simulink model "MPC_mobile_base_KIN_IPOPT_fast_ROS"  (R2018b)
settings: Solver=ode4  StartTime=0.0  StopTime=inf  FixedStep=Tsample  RelTol=1e-3
values from neighbouring files (symbols this model uses):
  initialize_starting_point = 1    [init_prova_vera1.mat]    (also in init_prova_vera3.mat; prova_vera1.mat = 0; prova_vera2.mat = 0)
  N = length(q)    [FK.m]    (also in FK_generation.m = size(DHTABLE,1); init_prova_vera1.mat = 10; init_prova_vera3.mat = 10; jacobian_MM.m)
  Np = 18    [init_prova_vera1.mat]    (also in init_prova_vera3.mat; initialization.m = Lf*2 + Lp*6; prova_vera1.mat; prova_vera2.mat)
  T = cell(N+1,1)    [FK.m]    (also in init_prova_vera1.mat = 0.5; init_prova_vera3.mat = 0.5; jacobian_MM.m; matlabultimo.mat = 0.5)
  Tsample = 0.01    [init_prova_vera1.mat]    (also in init_prova_vera3.mat; matlabultimo.mat; prova_vera1.mat; prova_vera2.mat)
  xd = [0 0 0 0 0 0 0 0 0 0.0238792670666 0.415141969475 1.22261425872 ... (1458 elements, 18x81)]    [init_prova_vera1.mat]    (also in init_prova_vera3.mat; liveplot.m = evalin('base','xd'); matlabultimo.mat = [0 0 0 0 0 0 0 0 0 -0.528285242967 -0.106449885857 1.3372295; prova_vera1.mat)
undefined symbols (not defined in the file or in its folder): Angular, Linear
libraries: robotlib x6, simulink x6, dspstat3 x3, peGeneralControl x1, sharedtransform x1
settings Model: EnablePacing=on  Creator=francesco  LastModifiedBy=francesco
settings ModelReferenceCC: PropagateVarSize=Only when enabling

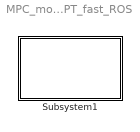
== system MPC_mobile_base_KIN_IPOPT_fast_ROS ==
  Subsystem1 : Subsystem  InitFcn=initialization

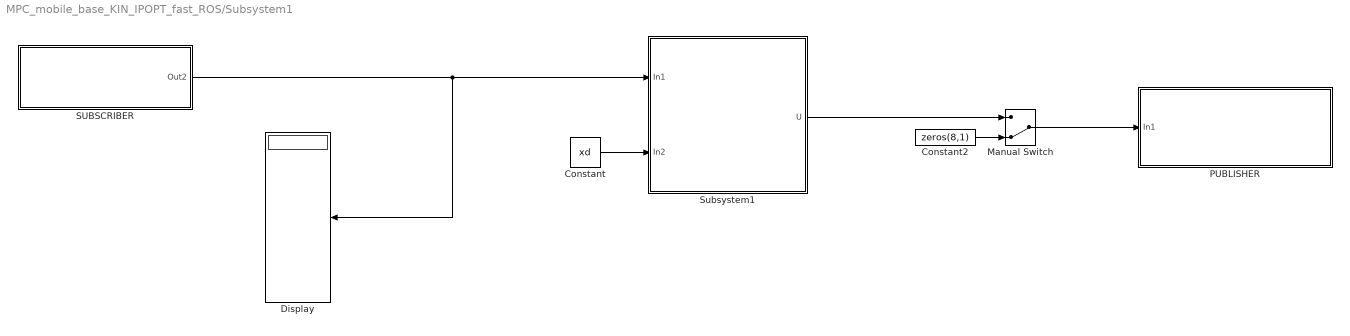
== system MPC_mobile_base_KIN_IPOPT_fast_ROS/Subsystem1 ==
  Constant : Constant  Value=xd
  Constant2 : Constant  Value=zeros(8,1)
  Display : Display
  Manual Switch : ManualSwitch  CurrentSetting=0
  PUBLISHER : Subsystem
  SUBSCRIBER : Subsystem
  Subsystem1 : Subsystem
      mask Display: fprintf('CONTROLLER')
  wires:
  Subsystem1/1(U) -> Manual Switch/1
  SUBSCRIBER/1(Out2) -> Subsystem1/1(In1), Display/1
  Constant/1 -> Subsystem1/2(In2)
  Constant2/1 -> Manual Switch/2
  Manual Switch/1 -> PUBLISHER/1(In1)

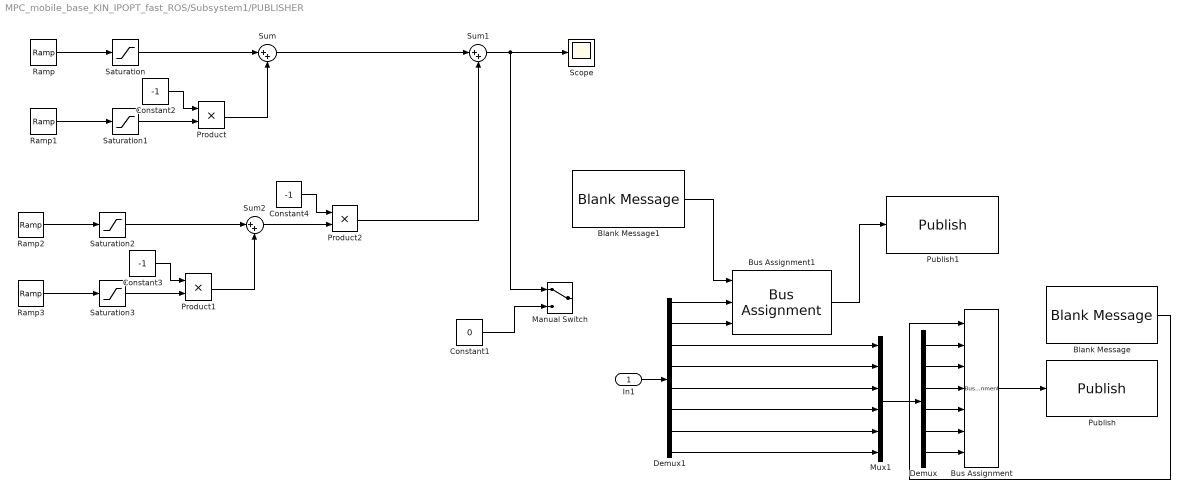
== system MPC_mobile_base_KIN_IPOPT_fast_ROS/Subsystem1/PUBLISHER ==
  In1 : Inport
  Blank Message : robotlib/Blank Message  messageClass=Message  entityType=geometry_msgs/Twist  messageType=geometry_msgs/Twist  SampleTime=inf
      settings: SourceProductBaseCode=RO
  Blank Message1 : robotlib/Blank Message  messageClass=Message  entityType=geometry_msgs/Twist  messageType=geometry_msgs/Twist  SampleTime=-1
      settings: SourceProductBaseCode=RO
  Bus Assignment : BusAssignment  AssignedSignals=Linear.X,Linear.Y,Linear.Z,Angular.X,Angular.Y,Angular.Z
  Bus Assignment1 : BusAssignment  AssignedSignals=Linear.X,Angular.Z
  Constant1 : Constant  Value=0  SampleTime=Tsample
  Constant2 : Constant  Value=-1  SampleTime=-1
  Constant3 : Constant  Value=-1  SampleTime=-1
  Constant4 : Constant  Value=-1  SampleTime=-1
  Demux : Demux  Outputs=6
  Demux1 : Demux  Outputs=8
  Manual Switch : ManualSwitch
  Mux1 : Mux  Inputs=6
  Product : Product
  Product1 : Product
  Product2 : Product
  Publish : robotlib/Publish  topicSource=Select from ROS network  topic=/MM_joint_speed  messageType=geometry_msgs/Twist  messageQueueLength=1
      settings: SourceProductBaseCode=RO
  Publish1 : robotlib/Publish  topicSource=Select from ROS network  topic=/cmd_vel  messageType=geometry_msgs/Twist  messageQueueLength=1
      settings: SourceProductBaseCode=RO
  Ramp : simulink/Sources/Ramp  slope=0.15  start=1  InitialOutput=0
  Ramp1 : simulink/Sources/Ramp  slope=0.15  start=12  InitialOutput=0
  Ramp2 : simulink/Sources/Ramp  slope=0.15  start=25  InitialOutput=0
  Ramp3 : simulink/Sources/Ramp  slope=0.15  start=35  InitialOutput=0
  Saturation{,1..3} (4 alike) : Saturate  UpperLimit=0.15  LowerLimit=-0.15
  Scope : Scope
  Sum : Sum  Inputs=|++
  Sum1 : Sum  Inputs=|++
  Sum2 : Sum  Inputs=|++
  wires:
  Demux/2 -> Bus Assignment/3
  Demux/3 -> Bus Assignment/4
  Demux/5 -> Bus Assignment/6
  Blank Message/1 -> Bus Assignment/1
  Demux/1 -> Bus Assignment/2
  Demux/6 -> Bus Assignment/7
  Bus Assignment/1 -> Publish/1
  Demux/4 -> Bus Assignment/5
  Demux1/3 -> Mux1/1
  Demux1/5 -> Mux1/3
  Demux1/8 -> Mux1/6
  Mux1/1 -> Demux/1
  Demux1/6 -> Mux1/4
  Demux1/7 -> Mux1/5
  In1/1 -> Demux1/1
  Demux1/4 -> Mux1/2
  Bus Assignment1/1 -> Publish1/1
  Blank Message1/1 -> Bus Assignment1/1
  Constant1/1 -> Manual Switch/2
  Ramp/1 -> Saturation/1
  Ramp1/1 -> Saturation1/1
  Saturation1/1 -> Product/2
  Constant2/1 -> Product/1
  Saturation/1 -> Sum/1
  Product/1 -> Sum/2
  Sum/1 -> Sum1/1
  Sum1/1 -> Manual Switch/1, Scope/1
  Ramp3/1 -> Saturation3/1
  Ramp2/1 -> Saturation2/1
  Saturation3/1 -> Product1/2
  Product1/1 -> Sum2/2
  Constant3/1 -> Product1/1
  Saturation2/1 -> Sum2/1
  Constant4/1 -> Product2/1
  Sum2/1 -> Product2/2
  Product2/1 -> Sum1/2
  Demux1/1 -> Bus Assignment1/2
  Demux1/2 -> Bus Assignment1/3

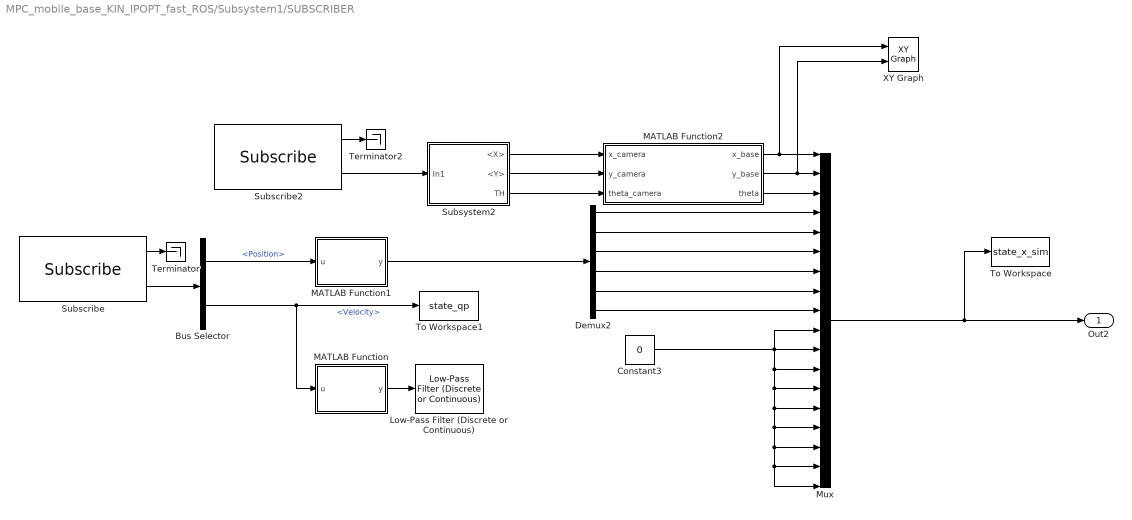
== system MPC_mobile_base_KIN_IPOPT_fast_ROS/Subsystem1/SUBSCRIBER ==
  Bus Selector : BusSelector  OutputSignals=Position,Velocity
  Constant3 : Constant  Value=0
  Demux2 : Demux  Outputs=6
  Low-Pass Filter (Discrete or Continuous) : peGeneralControl/Low-Pass Filter (Discrete or Continuous)  K=1  T=10  B=inf  A=-inf  Ts=-1
  MATLAB Function : MATLAB Function  TreatAsAtomicUnit=on
  MATLAB Function1 : MATLAB Function  TreatAsAtomicUnit=on
  MATLAB Function2 : MATLAB Function  TreatAsAtomicUnit=on
  Mux : Mux  Inputs=18
  Subscribe : robotlib/Subscribe  topicSource=Select from ROS network  topic=/joint_states  messageType=sensor_msgs/JointState  sampleTime=-1  messageQueueLength=1
      settings: SourceProductBaseCode=RO
  Subscribe2 : robotlib/Subscribe  topicSource=Select from ROS network  topic=/MM_base_pose  messageType=geometry_msgs/Pose  sampleTime=Tsample  messageQueueLength=1
      settings: SourceProductBaseCode=RO
  Subsystem2 : Subsystem
  Terminator : Terminator
  Terminator2 : Terminator
  To Workspace : ToWorkspace  VariableName=state_x_sim  SampleTime=T
  To Workspace1 : ToWorkspace  VariableName=state_qp  SampleTime=T
  XY Graph : simulink/Sinks/XY Graph  xmin=-1  xmax=10  ymin=-1  ymax=4  st=-1
  Out2 : Outport
  wires:
  Demux2/1 -> Mux/4
  Demux2/4 -> Mux/7
  Demux2/5 -> Mux/8
  Demux2/3 -> Mux/6
  MATLAB Function/1(y) -> Low-Pass Filter (Discrete or Continuous)/1
  Mux/1 -> To Workspace/1, Out2/1
  Demux2/2 -> Mux/5
  Bus Selector/1 -> MATLAB Function1/1(u)  "<Position>"
  Constant3/1 -> Mux/14, Mux/18, Mux/17, Mux/16, Mux/15, Mux/13, Mux/12, Mux/11, Mux/10
  Bus Selector/2 -> MATLAB Function/1(u), To Workspace1/1  "<Velocity>"
  Demux2/6 -> Mux/9
  Subscribe/2 -> Bus Selector/1
  MATLAB Function1/1(y) -> Demux2/1
  Subscribe/1 -> Terminator/1
  Subscribe2/1 -> Terminator2/1
  Subscribe2/2 -> Subsystem2/1(In1)
  MATLAB Function2/3(theta) -> Mux/3
  Subsystem2/3(TH) -> MATLAB Function2/3(theta_camera)
  Subsystem2/2(<Y>) -> MATLAB Function2/2(y_camera)
  Subsystem2/1(<X>) -> MATLAB Function2/1(x_camera)
  MATLAB Function2/2(y_base) -> Mux/2, XY Graph/2
  MATLAB Function2/1(x_base) -> Mux/1, XY Graph/1

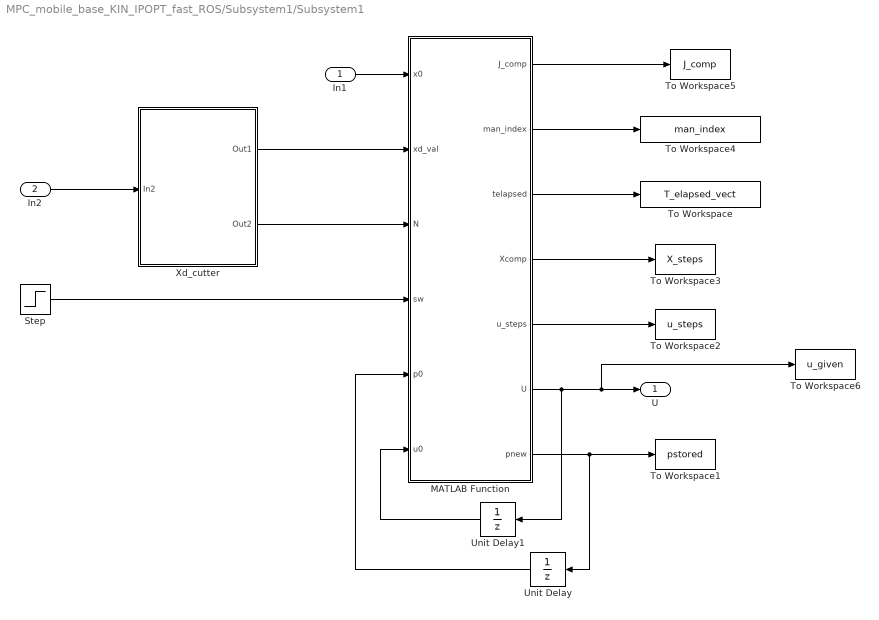
== system MPC_mobile_base_KIN_IPOPT_fast_ROS/Subsystem1/Subsystem1 ==
  In1 : Inport
  In2 : Inport  Port=2
  MATLAB Function : MATLAB Function  TreatAsAtomicUnit=on
  Step : Step  Time=0  SampleTime=0
  To Workspace : ToWorkspace  VariableName=T_elapsed_vect  SampleTime=T
  To Workspace1 : ToWorkspace  VariableName=pstored  SampleTime=-1
  To Workspace2 : ToWorkspace  VariableName=u_steps  SaveFormat=Structure  SampleTime=-1
  To Workspace3 : ToWorkspace  VariableName=X_steps  SaveFormat=Structure  SampleTime=-1
  To Workspace4 : ToWorkspace  VariableName=man_index  SampleTime=T
  To Workspace5 : ToWorkspace  VariableName=J_comp  SampleTime=-1
  To Workspace6 : ToWorkspace  VariableName=u_given  SampleTime=-1
  Unit Delay : UnitDelay  InitialCondition=zeros(Np,1)  SampleTime=T
  Unit Delay1 : UnitDelay  InitialCondition=zeros(8,1)  SampleTime=T
  Xd_cutter : Subsystem
  U : Outport  SampleTime=Tsample
  wires:
  MATLAB Function/7(pnew) -> To Workspace1/1, Unit Delay/1
  In1/1 -> MATLAB Function/1(x0)
  Unit Delay/1 -> MATLAB Function/5(p0)
  MATLAB Function/3(telapsed) -> To Workspace/1
  Unit Delay1/1 -> MATLAB Function/6(u0)
  MATLAB Function/5(u_steps) -> To Workspace2/1
  MATLAB Function/4(Xcomp) -> To Workspace3/1
  In2/1 -> Xd_cutter/1(In2)
  Xd_cutter/1(Out1) -> MATLAB Function/2(xd_val)
  Xd_cutter/2(Out2) -> MATLAB Function/3(N)
  Step/1 -> MATLAB Function/4(sw)
  MATLAB Function/2(man_index) -> To Workspace4/1
  MATLAB Function/1(J_comp) -> To Workspace5/1
  MATLAB Function/6(U) -> Unit Delay1/1, To Workspace6/1, U/1

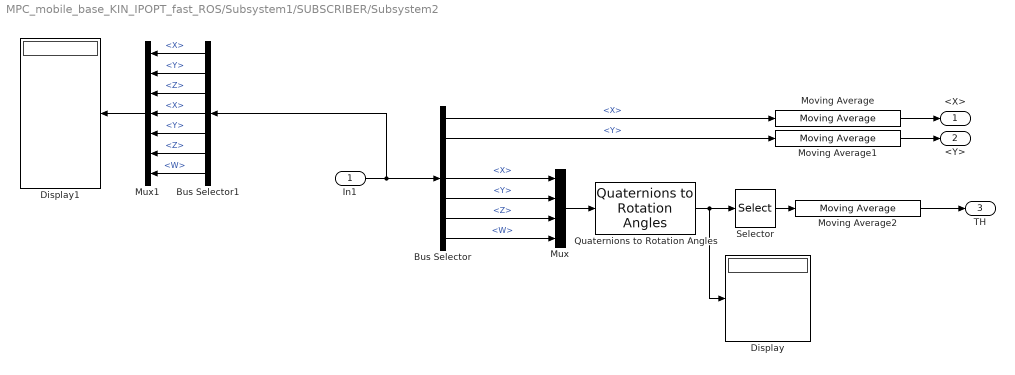
== system MPC_mobile_base_KIN_IPOPT_fast_ROS/Subsystem1/SUBSCRIBER/Subsystem2 ==
  In1 : Inport
  Bus Selector : BusSelector  OutputSignals=Position.X,Position.Y,Position.Z,Orientation.X,Orientation.Y,Orientation.Z,Orientation.W
  Bus Selector1 : BusSelector  OutputSignals=Position.X,Position.Y,Position.Z,Orientation.X,Orientation.Y,Orientation.Z,Orientation.W
  Display : Display
  Display1 : Display
  Moving Average : dspstat3/Moving Average  Method=Sliding window  ForgettingFactorPort=off  SpecifyWindowLength=on  WindowLength=5  ForgettingFactor=0.9  SimulateUsing=Code generation
  Moving Average1 : dspstat3/Moving Average  Method=Sliding window  ForgettingFactorPort=off  SpecifyWindowLength=on  WindowLength=5  ForgettingFactor=0.9  SimulateUsing=Code generation
  Moving Average2 : dspstat3/Moving Average  Method=Sliding window  ForgettingFactorPort=off  SpecifyWindowLength=on  WindowLength=5  ForgettingFactor=0.9  SimulateUsing=Code generation
  Mux : Mux
  Mux1 : Mux  Inputs=7
  Quaternions to Rotation Angles : sharedtransform/Quaternions to Rotation Angles  rotationOrder=ZYX  aMode=aMode
      settings: SourceProductBaseCode=AE
  Selector : Selector  InputPortWidth=3  IndexOptions=Index vector (dialog)  Indices=3  OutputSizes=1
  <X> : Outport
  <Y> : Outport  Port=2
  TH : Outport  Port=3
  wires:
  In1/1 -> Bus Selector1/1, Bus Selector/1
  Bus Selector/2 -> Moving Average1/1  "<Y>"
  Mux/1 -> Quaternions to Rotation Angles/1
  Quaternions to Rotation Angles/1 -> Selector/1, Display/1
  Bus Selector/1 -> Moving Average/1  "<X>"
  Bus Selector/7 -> Mux/4  "<W>"
  Bus Selector/6 -> Mux/3  "<Z>"
  Bus Selector/5 -> Mux/2  "<Y>"
  Bus Selector/4 -> Mux/1  "<X>"
  Bus Selector1/1 -> Mux1/1  "<X>"
  Bus Selector1/2 -> Mux1/2  "<Y>"
  Bus Selector1/3 -> Mux1/3  "<Z>"
  Bus Selector1/4 -> Mux1/4  "<X>"
  Bus Selector1/5 -> Mux1/5  "<Y>"
  Bus Selector1/6 -> Mux1/6  "<Z>"
  Bus Selector1/7 -> Mux1/7  "<W>"
  Mux1/1 -> Display1/1
  Selector/1 -> Moving Average2/1
  Moving Average/1 -> <X>/1
  Moving Average1/1 -> <Y>/1
  Moving Average2/1 -> TH/1

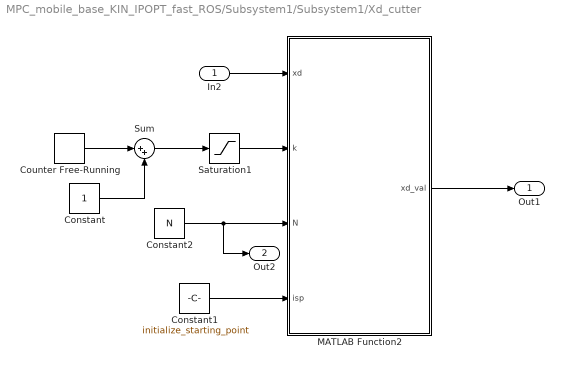
== system MPC_mobile_base_KIN_IPOPT_fast_ROS/Subsystem1/Subsystem1/Xd_cutter ==
  In2 : Inport
  Constant : Constant
  Constant1 : Constant  Value=initialize_starting_point
  Constant2 : Constant  Value=N
  Counter Free-Running : simulink/Sources/Counter Free-Running  NumBits=12  tsamp=T
  MATLAB Function2 : MATLAB Function  TreatAsAtomicUnit=on
  Saturation1 : Saturate  UpperLimit=size(xd,2)
  Sum : Sum  Inputs=|++
  Out1 : Outport
  Out2 : Outport  Port=2
  wires:
  Counter Free-Running/1 -> Sum/1
  Saturation1/1 -> MATLAB Function2/2(k)
  MATLAB Function2/1(xd_val) -> Out1/1
  Sum/1 -> Saturation1/1
  Constant/1 -> Sum/2
  Constant2/1 -> MATLAB Function2/3(N), Out2/1
  In2/1 -> MATLAB Function2/1(xd)
  Constant1/1 -> MATLAB Function2/4(isp)

== matlab function MPC_mobile_base_KIN_IPOPT_fast_ROS/Subsystem1/SUBSCRIBER/MATLAB Function ==
  data: u input; y output
function y = fcn(u)

y = u(1:6);

== matlab function MPC_mobile_base_KIN_IPOPT_fast_ROS/Subsystem1/Subsystem1/MATLAB Function ==
  settings: updateMethod=DISCRETE  sampleTime=T
  data: J_comp output; man_index output size=[1]; telapsed output; Xcomp output size=[18,N+1]; u_steps output size=[8,N]; U output; x0 input; pnew output; xd_val input; N input; sw input; p0 input; u0 input
function [J_comp,man_index,telapsed,Xcomp,u_steps,U,pnew] = fnc(x0,xd_val,N,sw,p0,u0)

coder.extrinsic('solver_NLP');
coder.extrinsic('evalin');
J_comp=zeros(1,6);

% INITIALIZING VARIABLES
telapsed=0;
u_steps=zeros(2,N);
pnew=zeros(size(p0));
U=zeros(8,1);
Xcomp=zeros(18,N);
man_index=0;

% SOLVING THE PROBLEM

[pnew, U, u_steps, Xcomp, telapsed, man, J_comp] = solver_NLP(xd_val,p0,x0,u0,sw);

man_index(1)=man;

end

== matlab function MPC_mobile_base_KIN_IPOPT_fast_ROS/Subsystem1/Subsystem1/Xd_cutter/MATLAB Function2 ==
  settings: updateMethod=DISCRETE  sampleTime=T
  data: xd input; k input; N input; xd_val output size=[18,N]; isp input
function xd_val = fcn(xd,k,N,isp)

    xd_val=zeros(18,N);

    if isp == 1
        xd_val=xd(:,1)*ones(1,N);
    else
        
        if size(xd,2)-k>N-1
        h=xd(:,k+1:k+N);

        else
        h=[xd(:,k+1:end) xd(:,end)*ones(1,N-(size(xd,2)-k))];

        end
    xd_val = h;

    end
end

== matlab function MPC_mobile_base_KIN_IPOPT_fast_ROS/Subsystem1/SUBSCRIBER/MATLAB Function1 ==
  data: u input; y output
function y = fcn(u)

y = u(1:6);

== matlab function MPC_mobile_base_KIN_IPOPT_fast_ROS/Subsystem1/SUBSCRIBER/MATLAB Function2 ==
  data: x_camera input; x_base output; y_camera input; theta_camera input; y_base output; theta output
function [x_base, y_base, theta] = fcn(x_camera,y_camera,theta_camera)

theta_marker  = -theta_camera;
x_marker = -y_camera;
y_marker = x_camera;


theta  = theta_marker+0.032; %rad
x_base = x_marker+0.695*cos(theta)+0.645;%-0.013*sin(theta);
y_base = y_marker+0.695*sin(theta)+1;%+0.013*cos(theta);
